simulink model "washingMachine"  (R2024b)
settings: Solver=VariableStepAuto  StartTime=0.0  StopTime=30.0  RelTol=1e-3
settings Model: Creator=optimus  LastModifiedBy=optimus

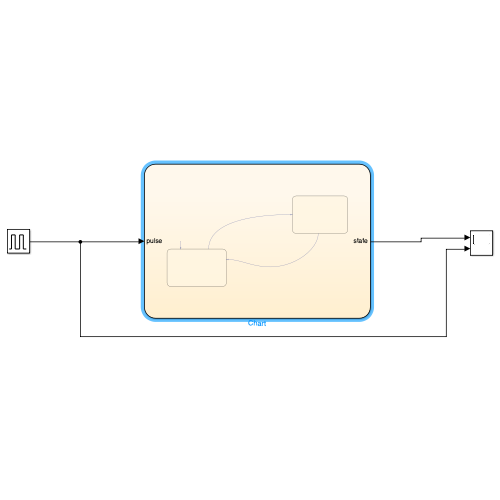
[thumbnail: Simulink's stored preview of the top-level diagram]
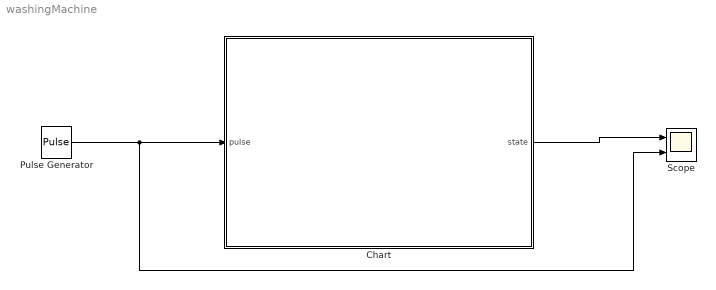
== system washingMachine ==
  Chart : Stateflow chart  TreatAsAtomicUnit=on
  Pulse Generator : DiscretePulseGenerator  PulseType=Time based  PulseWidth=50  PhaseDelay=1
  Scope : Scope  NumInputPorts=2
  wires:
  Pulse Generator/1 -> Scope/2, Chart/1(pulse)
  Chart/1(state) -> Scope/1

== stateflow chart washingMachine/Chart ==
  state Dirty_Washing
    entry:
    state=1;
    clean=0;
    during:
    clean=1;
  state Idle_Clean
    entry:
    state=0;
    load=0;
    during:
    load=1;
  Idle_Clean -> Dirty_Washing : after(2,sec)[pulse==1 && load==1]
  Dirty_Washing -> Idle_Clean : after(10,sec)[clean==1]
  (default) -> Idle_Clean
  data: pulse input; state output; clean local =0; load local =0
